simulink model "ultrasonido"  (R2018b)
settings: Solver=FixedStepDiscrete  StartTime=0.0  StopTime=20.0  FixedStep=0.01  RelTol=1e-3
undefined symbols (not defined in the file or in its folder): motorIp, motorSp
libraries: mobileRoboticsTrainingLib x5
settings Model: Creator=Juan David Gómez  LastModifiedBy=Juan David Gómez

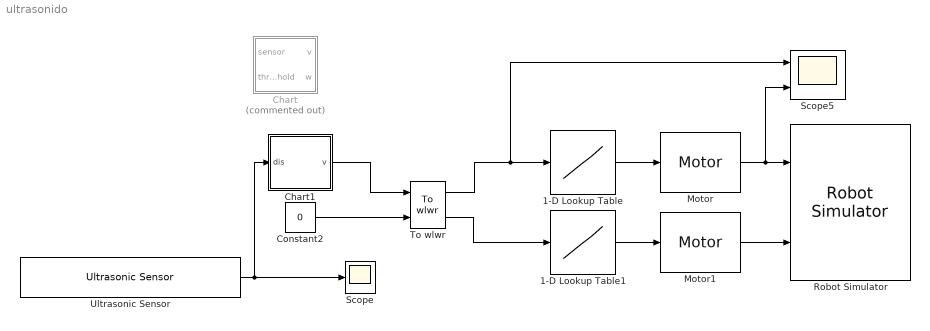
== system ultrasonido ==
  1-D Lookup Table : Lookup_n-D  NumberOfTableDimensions=1  BreakpointsForDimension1=motorSp  Table=motorIp  InternalRulePriority=Speed  RndMeth=Simplest  InputSameDT=on
  1-D Lookup Table1 : Lookup_n-D  NumberOfTableDimensions=1  BreakpointsForDimension1=motorSp  Table=motorIp  InternalRulePriority=Speed  RndMeth=Simplest  InputSameDT=on
  Chart : Stateflow chart  Commented=on  TreatAsAtomicUnit=on
  Chart1 : Stateflow chart  TreatAsAtomicUnit=on
  Constant2 : Constant  Value=0
  Motor : mobileRoboticsTrainingLib/Motor  motorPlant=wheelMotorModel  sensorType=Speed
      settings: SourceProductName=Mobile Robotics Training Library
  Motor1 : mobileRoboticsTrainingLib/Motor  motorPlant=wheelMotorModel  sensorType=Speed
      settings: SourceProductName=Mobile Robotics Training Library
  Robot Simulator : mobileRoboticsTrainingLib/Robot Simulator  Priority=99  mapVar=mapForSim  startX=0.051843  startY=0.76208  startTheta=0  axleLength=0.15  wheelR=0.03
  Scope : Scope
  Scope5 : Scope  NumInputPorts=2
  To wlwr : mobileRoboticsTrainingLib/To wlwr  axleLength=0.15  wheelR=0.03
  Ultrasonic Sensor : mobileRoboticsTrainingLib/Ultrasonic Sensor  mapVar=mapForSim  maxSenRange=2  minSenRange=0.02  senRes=0.01  sensOff=[0.15 0]
      settings: SourceProductName=Mobile Robotics Training Library
  wires:
  Motor/1 -> Scope5/2, Robot Simulator/1
  Motor1/1 -> Robot Simulator/2
  To wlwr/1 -> Scope5/1, 1-D Lookup Table/1
  1-D Lookup Table/1 -> Motor/1
  1-D Lookup Table1/1 -> Motor1/1
  To wlwr/2 -> 1-D Lookup Table1/1
  Constant2/1 -> To wlwr/2
  Ultrasonic Sensor/1 -> Chart1/1(dis), Scope/1
  Chart1/1(v) -> To wlwr/1

== stateflow chart ultrasonido/Chart1 ==
  state Avanzar
    v = 0.1;
  state pare
    v= 0;
  (default) -> Avanzar
  Avanzar -> pare : [v == 0.1 && 0.02< dis &&  dis < 0.1 ]
  data: dis input; v output

== stateflow chart ultrasonido/Chart ==
  state GiroDer
    v = 0.1
    w = -1
  state GiroIzq
    v = 0.1
    w = 1
  (default) -> GiroDer
  GiroDer -> GiroIzq : [sensor < threshold]
  GiroIzq -> GiroDer : [sensor >= threshold]
  data: sensor input; threshold input; v output; w output
